simulink model "Lineardigital"  (R2018a)
settings: Solver=VariableStepAuto  StartTime=0.0  StopTime=2  RelTol=1e-3
values from neighbouring files (symbols this model uses):
  pole1 = double(poles(2))    [Linearization&MDPP.m]
  pole2 = double(poles(3))    [Linearization&MDPP.m]
  rd = cell2mat(rdd)    [Linearization&MDPP.m]
  sd = cell2mat(sdd)    [Linearization&MDPP.m]
  td = cell2mat(tdd)    [Linearization&MDPP.m]
  Ts = 0.005*2*pi/fb    [Linearization&MDPP.m]
undefined symbols (not defined in the file or in its folder): b
settings Model: Creator=Hirsa  LastModifiedBy=Hirsa

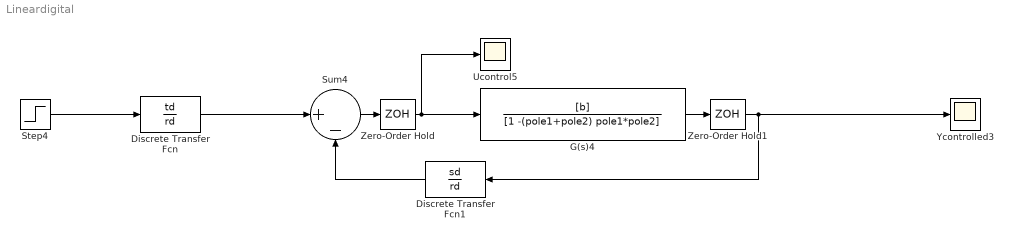
== system Lineardigital ==
  Discrete Transfer Fcn : DiscreteTransferFcn  Numerator=td  Denominator=rd  SampleTime=Ts
  Discrete Transfer Fcn1 : DiscreteTransferFcn  Numerator=sd  Denominator=rd  SampleTime=Ts
  G(s)4 : TransferFcn  Numerator=[b]  Denominator=[1 -(pole1+pole2) pole1*pole2]
  Step4 : Step
  Sum4 : Sum  Inputs=|+-
  Ucontrol5 : Scope
  Ycontrolled3 : Scope
  Zero-Order Hold : ZeroOrderHold  SampleTime=Ts
  Zero-Order Hold1 : ZeroOrderHold  SampleTime=Ts
  wires:
  Discrete Transfer Fcn1/1 -> Sum4/2
  Discrete Transfer Fcn/1 -> Sum4/1
  Sum4/1 -> Zero-Order Hold/1
  G(s)4/1 -> Zero-Order Hold1/1
  Step4/1 -> Discrete Transfer Fcn/1
  Zero-Order Hold/1 -> Ucontrol5/1, G(s)4/1
  Zero-Order Hold1/1 -> Discrete Transfer Fcn1/1, Ycontrolled3/1
